simulink model "VCU_CS75_12_16_Test"  (R2014a)
settings: Solver=FixedStepDiscrete  StartTime=0.0  StopTime=25  FixedStep=0.0005  RelTol=1e-3
undefined symbols (not defined in the file): ecucoder_acal, I_SW01_L, LaterlAngleCommand, LDW, RemoteAcclPosition
libraries: simulink x913, ec5744lib x39
(part 5 of 30)

== system VCU_CS75_12_16_Test/长安CS75底盘程序，20ms一次/Input/DBC转化的messages（存底）/ReceiveMessages13/SAS_108 ==
  input : Inport
  Demux : Demux  Outputs=8
  SAS_CRCCheck_Ad : Sum
  SAS_CRCCheck_Convert : DataTypeConversion  OutDataTypeStr=uint32
  SAS_CRCCheck_F : Gain
  SAS_CRCCheck_L : simulink/Logic and Bit Operations/Bitwise Operator  logicop=AND  UseBitMask=on  BitMask=255  BitMaskRealWorld=Stored Integer
  SAS_CRCCheck_O : Constant  Value=0  OutDataTypeStr=single
  SAS_CRCCheck_S : ArithShift
  SAS_CRCCheck_Sub : Subsystem
  SAS_CRCCheck_sat : Saturate  UpperLimit=255  LowerLimit=0
  SAS_CRCCheckcv : DataTypeConversion
  SAS_Calibrated_Ad : Sum
  SAS_Calibrated_Convert : DataTypeConversion  OutDataTypeStr=uint32
  SAS_Calibrated_F : Gain
  SAS_Calibrated_L : simulink/Logic and Bit Operations/Bitwise Operator  logicop=AND  UseBitMask=on  BitMask=32  BitMaskRealWorld=Stored Integer
  SAS_Calibrated_O : Constant  Value=0  OutDataTypeStr=single
  SAS_Calibrated_S : ArithShift  BitShiftNumber=5
  SAS_Calibrated_Sub : Subsystem
  SAS_Calibrated_sat : Saturate  UpperLimit=1  LowerLimit=0
  SAS_Calibratedcv : DataTypeConversion
  SAS_RollingCounter_Ad : Sum
  SAS_RollingCounter_Convert : DataTypeConversion  OutDataTypeStr=uint32
  SAS_RollingCounter_F : Gain
  SAS_RollingCounter_L : simulink/Logic and Bit Operations/Bitwise Operator  logicop=AND  UseBitMask=on  BitMask=15  BitMaskRealWorld=Stored Integer
  SAS_RollingCounter_O : Constant  Value=0  OutDataTypeStr=single
  SAS_RollingCounter_S : ArithShift
  SAS_RollingCounter_Sub : Subsystem
  SAS_RollingCounter_sat : Saturate  UpperLimit=15  LowerLimit=0
  SAS_RollingCountercv : DataTypeConversion
  SAS_SASFailure_Ad : Sum
  SAS_SASFailure_Convert : DataTypeConversion  OutDataTypeStr=uint32
  SAS_SASFailure_F : Gain
  SAS_SASFailure_L : simulink/Logic and Bit Operations/Bitwise Operator  logicop=AND  UseBitMask=on  BitMask=64  BitMaskRealWorld=Stored Integer
  SAS_SASFailure_O : Constant  Value=0  OutDataTypeStr=single
  SAS_SASFailure_S : ArithShift  BitShiftNumber=6
  SAS_SASFailure_Sub : Subsystem
  SAS_SASFailure_sat : Saturate  UpperLimit=1  LowerLimit=0
  SAS_SASFailurecv : DataTypeConversion
  SAS_SteeringAngleCS : ArithShift  BitShiftNumber=-16
  SAS_SteeringAngleCS1 : ArithShift  BitShiftNumber=-15
  SAS_SteeringAngleConS : Constant  OutDataTypeStr=single
  SAS_SteeringAngleMinus : UnaryMinus
  SAS_SteeringAngleROP : RelationalOperator  OutDataTypeStr=boolean
  SAS_SteeringAngleSW : Switch  Criteria=u2 ~= 0
  SAS_SteeringAngleSpeed_Ad : Sum
  SAS_SteeringAngleSpeed_Convert : DataTypeConversion  OutDataTypeStr=uint32
  SAS_SteeringAngleSpeed_F : Gain  Gain=4
  SAS_SteeringAngleSpeed_L : simulink/Logic and Bit Operations/Bitwise Operator  logicop=AND  UseBitMask=on  BitMask=255  BitMaskRealWorld=Stored Integer
  SAS_SteeringAngleSpeed_O : Constant  Value=0  OutDataTypeStr=single
  SAS_SteeringAngleSpeed_S : ArithShift
  SAS_SteeringAngleSpeed_Sub : Subsystem
  SAS_SteeringAngleSpeed_sat : Saturate  UpperLimit=1020  LowerLimit=0
  SAS_SteeringAngleSpeedcv : DataTypeConversion
  SAS_SteeringAngleValid_Ad : Sum
  SAS_SteeringAngleValid_Convert : DataTypeConversion  OutDataTypeStr=uint32
  SAS_SteeringAngleValid_F : Gain
  SAS_SteeringAngleValid_L : simulink/Logic and Bit Operations/Bitwise Operator  logicop=AND  UseBitMask=on  BitMask=128  BitMaskRealWorld=Stored Integer
  SAS_SteeringAngleValid_O : Constant  Value=0  OutDataTypeStr=single
  SAS_SteeringAngleValid_S : ArithShift  BitShiftNumber=7
  SAS_SteeringAngleValid_Sub : Subsystem
  SAS_SteeringAngleValid_sat : Saturate  UpperLimit=1  LowerLimit=0
  SAS_SteeringAngleValidcv : DataTypeConversion
  SAS_SteeringAngle_Ad : Sum
  SAS_SteeringAngle_Convert : DataTypeConversion  OutDataTypeStr=uint32
  SAS_SteeringAngle_F : Gain  Gain=0.1
  SAS_SteeringAngle_L : simulink/Logic and Bit Operations/Bitwise Operator  logicop=AND  UseBitMask=on  BitMask=65535  BitMaskRealWorld=Stored Integer
  SAS_SteeringAngle_O : Constant  Value=0  OutDataTypeStr=single
  SAS_SteeringAngle_S : ArithShift
  SAS_SteeringAngle_Sub : Subsystem
  SAS_SteeringAngle_sat : Saturate  UpperLimit=780  LowerLimit=-780
  SAS_SteeringAnglecv : DataTypeConversion
  SAS_SteeringAngleinput1_Ad : Sum
  SAS_SteeringAngleinput1_C : Constant  Value=256
  SAS_SteeringAngleinput1_P : Product
  SAS_SteeringAnglesubcon : Sum  Inputs=+-
  SAS_SteeringAngle_Out : Outport
  SAS_SteeringAngleSpeed_Out : Outport  Port=2
  SAS_Calibrated_Out : Outport  Port=3
  SAS_SASFailure_Out : Outport  Port=4
  SAS_SteeringAngleValid_Out : Outport  Port=5
  SAS_RollingCounter_Out : Outport  Port=6
  SAS_CRCCheck_Out : Outport  Port=7
  wires:
  input/1 -> Demux/1
  SAS_CRCCheckcv/1 -> SAS_CRCCheck_F/1
  SAS_CRCCheck_S/1 -> SAS_CRCCheckcv/1
  SAS_CRCCheck_L/1 -> SAS_CRCCheck_S/1
  SAS_CRCCheck_Convert/1 -> SAS_CRCCheck_L/1
  SAS_CRCCheck_Sub/1(Out1) -> SAS_CRCCheck_Convert/1
  Demux/8 -> SAS_CRCCheck_Sub/1(In1)
  SAS_CRCCheck_sat/1 -> SAS_CRCCheck_Out/1
  SAS_CRCCheck_Ad/1 -> SAS_CRCCheck_sat/1
  SAS_CRCCheck_O/1 -> SAS_CRCCheck_Ad/2
  SAS_CRCCheck_F/1 -> SAS_CRCCheck_Ad/1
  SAS_RollingCountercv/1 -> SAS_RollingCounter_F/1
  SAS_RollingCounter_S/1 -> SAS_RollingCountercv/1
  SAS_RollingCounter_L/1 -> SAS_RollingCounter_S/1
  SAS_RollingCounter_Convert/1 -> SAS_RollingCounter_L/1
  SAS_RollingCounter_Sub/1(Out1) -> SAS_RollingCounter_Convert/1
  Demux/7 -> SAS_RollingCounter_Sub/1(In1)
  SAS_RollingCounter_sat/1 -> SAS_RollingCounter_Out/1
  SAS_RollingCounter_Ad/1 -> SAS_RollingCounter_sat/1
  SAS_RollingCounter_O/1 -> SAS_RollingCounter_Ad/2
  SAS_RollingCounter_F/1 -> SAS_RollingCounter_Ad/1
  SAS_SteeringAngleValidcv/1 -> SAS_SteeringAngleValid_F/1
  SAS_SteeringAngleValid_S/1 -> SAS_SteeringAngleValidcv/1
  SAS_SteeringAngleValid_L/1 -> SAS_SteeringAngleValid_S/1
  SAS_SteeringAngleValid_Convert/1 -> SAS_SteeringAngleValid_L/1
  SAS_SteeringAngleValid_Sub/1(Out1) -> SAS_SteeringAngleValid_Convert/1
  SAS_SteeringAngleValid_sat/1 -> SAS_SteeringAngleValid_Out/1
  SAS_SteeringAngleValid_Ad/1 -> SAS_SteeringAngleValid_sat/1
  SAS_SteeringAngleValid_O/1 -> SAS_SteeringAngleValid_Ad/2
  SAS_SteeringAngleValid_F/1 -> SAS_SteeringAngleValid_Ad/1
  SAS_SASFailurecv/1 -> SAS_SASFailure_F/1
  SAS_SASFailure_S/1 -> SAS_SASFailurecv/1
  SAS_SASFailure_L/1 -> SAS_SASFailure_S/1
  SAS_SASFailure_Convert/1 -> SAS_SASFailure_L/1
  SAS_SASFailure_Sub/1(Out1) -> SAS_SASFailure_Convert/1
  SAS_SASFailure_sat/1 -> SAS_SASFailure_Out/1
  SAS_SASFailure_Ad/1 -> SAS_SASFailure_sat/1
  SAS_SASFailure_O/1 -> SAS_SASFailure_Ad/2
  SAS_SASFailure_F/1 -> SAS_SASFailure_Ad/1
  SAS_Calibratedcv/1 -> SAS_Calibrated_F/1
  SAS_Calibrated_S/1 -> SAS_Calibratedcv/1
  SAS_Calibrated_L/1 -> SAS_Calibrated_S/1
  SAS_Calibrated_Convert/1 -> SAS_Calibrated_L/1
  SAS_Calibrated_Sub/1(Out1) -> SAS_Calibrated_Convert/1
  Demux/4 -> SAS_SteeringAngleValid_Sub/1(In1), SAS_SASFailure_Sub/1(In1), SAS_Calibrated_Sub/1(In1)
  SAS_Calibrated_sat/1 -> SAS_Calibrated_Out/1
  SAS_Calibrated_Ad/1 -> SAS_Calibrated_sat/1
  SAS_Calibrated_O/1 -> SAS_Calibrated_Ad/2
  SAS_Calibrated_F/1 -> SAS_Calibrated_Ad/1
  SAS_SteeringAngleSpeedcv/1 -> SAS_SteeringAngleSpeed_F/1
  SAS_SteeringAngleSpeed_S/1 -> SAS_SteeringAngleSpeedcv/1
  SAS_SteeringAngleSpeed_L/1 -> SAS_SteeringAngleSpeed_S/1
  SAS_SteeringAngleSpeed_Convert/1 -> SAS_SteeringAngleSpeed_L/1
  SAS_SteeringAngleSpeed_Sub/1(Out1) -> SAS_SteeringAngleSpeed_Convert/1
  Demux/3 -> SAS_SteeringAngleSpeed_Sub/1(In1)
  SAS_SteeringAngleSpeed_sat/1 -> SAS_SteeringAngleSpeed_Out/1
  SAS_SteeringAngleSpeed_Ad/1 -> SAS_SteeringAngleSpeed_sat/1
  SAS_SteeringAngleSpeed_O/1 -> SAS_SteeringAngleSpeed_Ad/2
  SAS_SteeringAngleSpeed_F/1 -> SAS_SteeringAngleSpeed_Ad/1
  SAS_SteeringAngleROP/1 -> SAS_SteeringAngleSW/2
  SAS_SteeringAngleSW/1 -> SAS_SteeringAngle_F/1
  SAS_SteeringAngleMinus/1 -> SAS_SteeringAngleSW/1
  SAS_SteeringAnglesubcon/1 -> SAS_SteeringAngleMinus/1
  SAS_SteeringAngleCS/1 -> SAS_SteeringAnglesubcon/1
  SAS_SteeringAngleCS1/1 -> SAS_SteeringAngleROP/2
  SAS_SteeringAngleConS/1 -> SAS_SteeringAngleCS1/1, SAS_SteeringAngleCS/1
  SAS_SteeringAnglecv/1 -> SAS_SteeringAngleSW/3, SAS_SteeringAnglesubcon/2, SAS_SteeringAngleROP/1
  SAS_SteeringAngle_S/1 -> SAS_SteeringAnglecv/1
  SAS_SteeringAngle_L/1 -> SAS_SteeringAngle_S/1
  SAS_SteeringAngle_Convert/1 -> SAS_SteeringAngle_L/1
  SAS_SteeringAngle_Sub/1(Out1) -> SAS_SteeringAngle_Convert/1
  SAS_SteeringAngleinput1_Ad/1 -> SAS_SteeringAngle_Sub/1(In1)
  Demux/2 -> SAS_SteeringAngleinput1_Ad/2
  SAS_SteeringAngleinput1_P/1 -> SAS_SteeringAngleinput1_Ad/1
  SAS_SteeringAngleinput1_C/1 -> SAS_SteeringAngleinput1_P/2
  Demux/1 -> SAS_SteeringAngleinput1_P/1
  SAS_SteeringAngle_sat/1 -> SAS_SteeringAngle_Out/1
  SAS_SteeringAngle_Ad/1 -> SAS_SteeringAngle_sat/1
  SAS_SteeringAngle_O/1 -> SAS_SteeringAngle_Ad/2
  SAS_SteeringAngle_F/1 -> SAS_SteeringAngle_Ad/1

== system VCU_CS75_12_16_Test/长安CS75底盘程序，20ms一次/Input/DBC转化的messages（存底）/ReceiveMessages14/SCM_3B8 ==
  input : Inport
  Demux : Demux  Outputs=8
  SCM_ACCCancel_Ad : Sum
  SCM_ACCCancel_Convert : DataTypeConversion  OutDataTypeStr=uint32
  SCM_ACCCancel_F : Gain
  SCM_ACCCancel_L : simulink/Logic and Bit Operations/Bitwise Operator  logicop=AND  UseBitMask=on  BitMask=4  BitMaskRealWorld=Stored Integer
  SCM_ACCCancel_O : Constant  Value=0  OutDataTypeStr=single
  SCM_ACCCancel_S : ArithShift  BitShiftNumber=2
  SCM_ACCCancel_Sub : Subsystem
  SCM_ACCCancel_sat : Saturate  UpperLimit=0  LowerLimit=0
  SCM_ACCCancelcv : DataTypeConversion
  SCM_ACCOn_Ad : Sum
  SCM_ACCOn_Convert : DataTypeConversion  OutDataTypeStr=uint32
  SCM_ACCOn_F : Gain
  SCM_ACCOn_L : simulink/Logic and Bit Operations/Bitwise Operator  logicop=AND  UseBitMask=on  BitMask=1  BitMaskRealWorld=Stored Integer
  SCM_ACCOn_O : Constant  Value=0  OutDataTypeStr=single
  SCM_ACCOn_S : ArithShift
  SCM_ACCOn_Sub : Subsystem
  SCM_ACCOn_sat : Saturate  UpperLimit=0  LowerLimit=0
  SCM_ACCOncv : DataTypeConversion
  SCM_IACCOn_Ad : Sum
  SCM_IACCOn_Convert : DataTypeConversion  OutDataTypeStr=uint32
  SCM_IACCOn_F : Gain
  SCM_IACCOn_L : simulink/Logic and Bit Operations/Bitwise Operator  logicop=AND  UseBitMask=on  BitMask=16  BitMaskRealWorld=Stored Integer
  SCM_IACCOn_O : Constant  Value=0  OutDataTypeStr=single
  SCM_IACCOn_S : ArithShift  BitShiftNumber=4
  SCM_IACCOn_Sub : Subsystem
  SCM_IACCOn_sat : Saturate  UpperLimit=0  LowerLimit=0
  SCM_IACCOncv : DataTypeConversion
  SCM_Resume_Ad : Sum
  SCM_Resume_Convert : DataTypeConversion  OutDataTypeStr=uint32
  SCM_Resume_F : Gain
  SCM_Resume_L : simulink/Logic and Bit Operations/Bitwise Operator  logicop=AND  UseBitMask=on  BitMask=16  BitMaskRealWorld=Stored Integer
  SCM_Resume_O : Constant  Value=0  OutDataTypeStr=single
  SCM_Resume_S : ArithShift  BitShiftNumber=4
  SCM_Resume_Sub : Subsystem
  SCM_Resume_sat : Saturate  UpperLimit=0  LowerLimit=0
  SCM_Resumecv : DataTypeConversion
  SCM_Speeddecrease_Ad : Sum
  SCM_Speeddecrease_Convert : DataTypeConversion  OutDataTypeStr=uint32
  SCM_Speeddecrease_F : Gain
  SCM_Speeddecrease_L : simulink/Logic and Bit Operations/Bitwise Operator  logicop=AND  UseBitMask=on  BitMask=64  BitMaskRealWorld=Stored Integer
  SCM_Speeddecrease_O : Constant  Value=0  OutDataTypeStr=single
  SCM_Speeddecrease_S : ArithShift  BitShiftNumber=6
  SCM_Speeddecrease_Sub : Subsystem
  SCM_Speeddecrease_sat : Saturate  UpperLimit=0  LowerLimit=0
  SCM_Speeddecreasecv : DataTypeConversion
  SCM_TimeGap_Ad : Sum
  SCM_TimeGap_Convert : DataTypeConversion  OutDataTypeStr=uint32
  SCM_TimeGap_F : Gain
  SCM_TimeGap_L : simulink/Logic and Bit Operations/Bitwise Operator  logicop=AND  UseBitMask=on  BitMask=1  BitMaskRealWorld=Stored Integer
  SCM_TimeGap_O : Constant  Value=0  OutDataTypeStr=single
  SCM_TimeGap_S : ArithShift
  SCM_TimeGap_Sub : Subsystem
  SCM_TimeGap_sat : Saturate  UpperLimit=0  LowerLimit=0
  SCM_TimeGapcv : DataTypeConversion
  SCM_ACCOn_Out : Outport
  SCM_ACCCancel_Out : Outport  Port=2
  SCM_Resume_Out : Outport  Port=3
  SCM_Speeddecrease_Out : Outport  Port=4
  SCM_TimeGap_Out : Outport  Port=5
  SCM_IACCOn_Out : Outport  Port=6
  wires:
  input/1 -> Demux/1
  SCM_IACCOncv/1 -> SCM_IACCOn_F/1
  SCM_IACCOn_S/1 -> SCM_IACCOncv/1
  SCM_IACCOn_L/1 -> SCM_IACCOn_S/1
  SCM_IACCOn_Convert/1 -> SCM_IACCOn_L/1
  SCM_IACCOn_Sub/1(Out1) -> SCM_IACCOn_Convert/1
  SCM_IACCOn_sat/1 -> SCM_IACCOn_Out/1
  SCM_IACCOn_Ad/1 -> SCM_IACCOn_sat/1
  SCM_IACCOn_O/1 -> SCM_IACCOn_Ad/2
  SCM_IACCOn_F/1 -> SCM_IACCOn_Ad/1
  SCM_TimeGapcv/1 -> SCM_TimeGap_F/1
  SCM_TimeGap_S/1 -> SCM_TimeGapcv/1
  SCM_TimeGap_L/1 -> SCM_TimeGap_S/1
  SCM_TimeGap_Convert/1 -> SCM_TimeGap_L/1
  SCM_TimeGap_Sub/1(Out1) -> SCM_TimeGap_Convert/1
  Demux/2 -> SCM_IACCOn_Sub/1(In1), SCM_TimeGap_Sub/1(In1)
  SCM_TimeGap_sat/1 -> SCM_TimeGap_Out/1
  SCM_TimeGap_Ad/1 -> SCM_TimeGap_sat/1
  SCM_TimeGap_O/1 -> SCM_TimeGap_Ad/2
  SCM_TimeGap_F/1 -> SCM_TimeGap_Ad/1
  SCM_Speeddecreasecv/1 -> SCM_Speeddecrease_F/1
  SCM_Speeddecrease_S/1 -> SCM_Speeddecreasecv/1
  SCM_Speeddecrease_L/1 -> SCM_Speeddecrease_S/1
  SCM_Speeddecrease_Convert/1 -> SCM_Speeddecrease_L/1
  SCM_Speeddecrease_Sub/1(Out1) -> SCM_Speeddecrease_Convert/1
  SCM_Speeddecrease_sat/1 -> SCM_Speeddecrease_Out/1
  SCM_Speeddecrease_Ad/1 -> SCM_Speeddecrease_sat/1
  SCM_Speeddecrease_O/1 -> SCM_Speeddecrease_Ad/2
  SCM_Speeddecrease_F/1 -> SCM_Speeddecrease_Ad/1
  SCM_Resumecv/1 -> SCM_Resume_F/1
  SCM_Resume_S/1 -> SCM_Resumecv/1
  SCM_Resume_L/1 -> SCM_Resume_S/1
  SCM_Resume_Convert/1 -> SCM_Resume_L/1
  SCM_Resume_Sub/1(Out1) -> SCM_Resume_Convert/1
  SCM_Resume_sat/1 -> SCM_Resume_Out/1
  SCM_Resume_Ad/1 -> SCM_Resume_sat/1
  SCM_Resume_O/1 -> SCM_Resume_Ad/2
  SCM_Resume_F/1 -> SCM_Resume_Ad/1
  SCM_ACCCancelcv/1 -> SCM_ACCCancel_F/1
  SCM_ACCCancel_S/1 -> SCM_ACCCancelcv/1
  SCM_ACCCancel_L/1 -> SCM_ACCCancel_S/1
  SCM_ACCCancel_Convert/1 -> SCM_ACCCancel_L/1
  SCM_ACCCancel_Sub/1(Out1) -> SCM_ACCCancel_Convert/1
  SCM_ACCCancel_sat/1 -> SCM_ACCCancel_Out/1
  SCM_ACCCancel_Ad/1 -> SCM_ACCCancel_sat/1
  SCM_ACCCancel_O/1 -> SCM_ACCCancel_Ad/2
  SCM_ACCCancel_F/1 -> SCM_ACCCancel_Ad/1
  SCM_ACCOncv/1 -> SCM_ACCOn_F/1
  SCM_ACCOn_S/1 -> SCM_ACCOncv/1
  SCM_ACCOn_L/1 -> SCM_ACCOn_S/1
  SCM_ACCOn_Convert/1 -> SCM_ACCOn_L/1
  SCM_ACCOn_Sub/1(Out1) -> SCM_ACCOn_Convert/1
  Demux/1 -> SCM_Speeddecrease_Sub/1(In1), SCM_Resume_Sub/1(In1), SCM_ACCCancel_Sub/1(In1), SCM_ACCOn_Sub/1(In1)
  SCM_ACCOn_sat/1 -> SCM_ACCOn_Out/1
  SCM_ACCOn_Ad/1 -> SCM_ACCOn_sat/1
  SCM_ACCOn_O/1 -> SCM_ACCOn_Ad/2
  SCM_ACCOn_F/1 -> SCM_ACCOn_Ad/1

== system VCU_CS75_12_16_Test/长安CS75底盘程序，20ms一次/Input/DBC转化的messages（存底）/ReceiveMessages15/SRS_005 ==
  input : Inport
  Demux : Demux  Outputs=8
  SRS_DriverBuckleSwitchStatus_Ad : Sum
  SRS_DriverBuckleSwitchStatus_Convert : DataTypeConversion  OutDataTypeStr=uint32
  SRS_DriverBuckleSwitchStatus_F : Gain
  SRS_DriverBuckleSwitchStatus_L : simulink/Logic and Bit Operations/Bitwise Operator  logicop=AND  UseBitMask=on  BitMask=192  BitMaskRealWorld=Stored Integer
  SRS_DriverBuckleSwitchStatus_O : Constant  Value=0  OutDataTypeStr=single
  SRS_DriverBuckleSwitchStatus_S : ArithShift  BitShiftNumber=6
  SRS_DriverBuckleSwitchStatus_Sub : Subsystem
  SRS_DriverBuckleSwitchStatus_sat : Saturate  UpperLimit=3  LowerLimit=0
  SRS_DriverBuckleSwitchStatuscv : DataTypeConversion
  SRS_RollingCounter_Ad : Sum
  SRS_RollingCounter_Convert : DataTypeConversion  OutDataTypeStr=uint32
  SRS_RollingCounter_F : Gain
  SRS_RollingCounter_L : simulink/Logic and Bit Operations/Bitwise Operator  logicop=AND  UseBitMask=on  BitMask=15  BitMaskRealWorld=Stored Integer
  SRS_RollingCounter_O : Constant  Value=0  OutDataTypeStr=single
  SRS_RollingCounter_S : ArithShift
  SRS_RollingCounter_Sub : Subsystem
  SRS_RollingCounter_sat : Saturate  UpperLimit=15  LowerLimit=0
  SRS_RollingCountercv : DataTypeConversion
  SRS_DriverBuckleSwitchStatus_Out : Outport
  SRS_RollingCounter_Out : Outport  Port=2
  wires:
  input/1 -> Demux/1
  SRS_RollingCountercv/1 -> SRS_RollingCounter_F/1
  SRS_RollingCounter_S/1 -> SRS_RollingCountercv/1
  SRS_RollingCounter_L/1 -> SRS_RollingCounter_S/1
  SRS_RollingCounter_Convert/1 -> SRS_RollingCounter_L/1
  SRS_RollingCounter_Sub/1(Out1) -> SRS_RollingCounter_Convert/1
  Demux/4 -> SRS_RollingCounter_Sub/1(In1)
  SRS_RollingCounter_sat/1 -> SRS_RollingCounter_Out/1
  SRS_RollingCounter_Ad/1 -> SRS_RollingCounter_sat/1
  SRS_RollingCounter_O/1 -> SRS_RollingCounter_Ad/2
  SRS_RollingCounter_F/1 -> SRS_RollingCounter_Ad/1
  SRS_DriverBuckleSwitchStatuscv/1 -> SRS_DriverBuckleSwitchStatus_F/1
  SRS_DriverBuckleSwitchStatus_S/1 -> SRS_DriverBuckleSwitchStatuscv/1
  SRS_DriverBuckleSwitchStatus_L/1 -> SRS_DriverBuckleSwitchStatus_S/1
  SRS_DriverBuckleSwitchStatus_Convert/1 -> SRS_DriverBuckleSwitchStatus_L/1
  SRS_DriverBuckleSwitchStatus_Sub/1(Out1) -> SRS_DriverBuckleSwitchStatus_Convert/1
  Demux/2 -> SRS_DriverBuckleSwitchStatus_Sub/1(In1)
  SRS_DriverBuckleSwitchStatus_sat/1 -> SRS_DriverBuckleSwitchStatus_Out/1
  SRS_DriverBuckleSwitchStatus_Ad/1 -> SRS_DriverBuckleSwitchStatus_sat/1
  SRS_DriverBuckleSwitchStatus_O/1 -> SRS_DriverBuckleSwitchStatus_Ad/2
  SRS_DriverBuckleSwitchStatus_F/1 -> SRS_DriverBuckleSwitchStatus_Ad/1

== system VCU_CS75_12_16_Test/长安CS75底盘程序，20ms一次/Input/DBC转化的messages（存底）/ReceiveMessages16/TCU_286 ==
  input : Inport
  Demux : Demux  Outputs=8
  TCU_ActualGearValid_Ad : Sum
  TCU_ActualGearValid_Convert : DataTypeConversion  OutDataTypeStr=uint32
  TCU_ActualGearValid_F : Gain
  TCU_ActualGearValid_L : simulink/Logic and Bit Operations/Bitwise Operator  logicop=AND  UseBitMask=on  BitMask=32  BitMaskRealWorld=Stored Integer
  TCU_ActualGearValid_O : Constant  Value=0  OutDataTypeStr=single
  TCU_ActualGearValid_S : ArithShift  BitShiftNumber=5
  TCU_ActualGearValid_Sub : Subsystem
  TCU_ActualGearValid_sat : Saturate  UpperLimit=1  LowerLimit=0
  TCU_ActualGearValidcv : DataTypeConversion
  TCU_ActualGear_Ad : Sum
  TCU_ActualGear_Convert : DataTypeConversion  OutDataTypeStr=uint32
  TCU_ActualGear_F : Gain
  TCU_ActualGear_L : simulink/Logic and Bit Operations/Bitwise Operator  logicop=AND  UseBitMask=on  BitMask=15  BitMaskRealWorld=Stored Integer
  TCU_ActualGear_O : Constant  Value=0  OutDataTypeStr=single
  TCU_ActualGear_S : ArithShift
  TCU_ActualGear_Sub : Subsystem
  TCU_ActualGear_sat : Saturate  UpperLimit=15  LowerLimit=0
  TCU_ActualGearcv : DataTypeConversion
  TCU_GearShiftPosition_Ad : Sum
  TCU_GearShiftPosition_Convert : DataTypeConversion  OutDataTypeStr=uint32
  TCU_GearShiftPosition_F : Gain
  TCU_GearShiftPosition_L : simulink/Logic and Bit Operations/Bitwise Operator  logicop=AND  UseBitMask=on  BitMask=240  BitMaskRealWorld=Stored Integer
  TCU_GearShiftPosition_O : Constant  Value=0  OutDataTypeStr=single
  TCU_GearShiftPosition_S : ArithShift  BitShiftNumber=4
  TCU_GearShiftPosition_Sub : Subsystem
  TCU_GearShiftPosition_sat : Saturate  UpperLimit=15  LowerLimit=0
  TCU_GearShiftPositioncv : DataTypeConversion
  TCU_ShiftPositionValid_Ad : Sum
  TCU_ShiftPositionValid_Convert : DataTypeConversion  OutDataTypeStr=uint32
  TCU_ShiftPositionValid_F : Gain
  TCU_ShiftPositionValid_L : simulink/Logic and Bit Operations/Bitwise Operator  logicop=AND  UseBitMask=on  BitMask=16  BitMaskRealWorld=Stored Integer
  TCU_ShiftPositionValid_O : Constant  Value=0  OutDataTypeStr=single
  TCU_ShiftPositionValid_S : ArithShift  BitShiftNumber=4
  TCU_ShiftPositionValid_Sub : Subsystem
  TCU_ShiftPositionValid_sat : Saturate  UpperLimit=1  LowerLimit=0
  TCU_ShiftPositionValidcv : DataTypeConversion
  TCU_ActualGear_Out : Outport
  TCU_ShiftPositionValid_Out : Outport  Port=2
  TCU_ActualGearValid_Out : Outport  Port=3
  TCU_GearShiftPosition_Out : Outport  Port=4
  wires:
  input/1 -> Demux/1
  TCU_GearShiftPositioncv/1 -> TCU_GearShiftPosition_F/1
  TCU_GearShiftPosition_S/1 -> TCU_GearShiftPositioncv/1
  TCU_GearShiftPosition_L/1 -> TCU_GearShiftPosition_S/1
  TCU_GearShiftPosition_Convert/1 -> TCU_GearShiftPosition_L/1
  TCU_GearShiftPosition_Sub/1(Out1) -> TCU_GearShiftPosition_Convert/1
  Demux/3 -> TCU_GearShiftPosition_Sub/1(In1)
  TCU_GearShiftPosition_sat/1 -> TCU_GearShiftPosition_Out/1
  TCU_GearShiftPosition_Ad/1 -> TCU_GearShiftPosition_sat/1
  TCU_GearShiftPosition_O/1 -> TCU_GearShiftPosition_Ad/2
  TCU_GearShiftPosition_F/1 -> TCU_GearShiftPosition_Ad/1
  TCU_ActualGearValidcv/1 -> TCU_ActualGearValid_F/1
  TCU_ActualGearValid_S/1 -> TCU_ActualGearValidcv/1
  TCU_ActualGearValid_L/1 -> TCU_ActualGearValid_S/1
  TCU_ActualGearValid_Convert/1 -> TCU_ActualGearValid_L/1
  TCU_ActualGearValid_Sub/1(Out1) -> TCU_ActualGearValid_Convert/1
  TCU_ActualGearValid_sat/1 -> TCU_ActualGearValid_Out/1
  TCU_ActualGearValid_Ad/1 -> TCU_ActualGearValid_sat/1
  TCU_ActualGearValid_O/1 -> TCU_ActualGearValid_Ad/2
  TCU_ActualGearValid_F/1 -> TCU_ActualGearValid_Ad/1
  TCU_ShiftPositionValidcv/1 -> TCU_ShiftPositionValid_F/1
  TCU_ShiftPositionValid_S/1 -> TCU_ShiftPositionValidcv/1
  TCU_ShiftPositionValid_L/1 -> TCU_ShiftPositionValid_S/1
  TCU_ShiftPositionValid_Convert/1 -> TCU_ShiftPositionValid_L/1
  TCU_ShiftPositionValid_Sub/1(Out1) -> TCU_ShiftPositionValid_Convert/1
  TCU_ShiftPositionValid_sat/1 -> TCU_ShiftPositionValid_Out/1
  TCU_ShiftPositionValid_Ad/1 -> TCU_ShiftPositionValid_sat/1
  TCU_ShiftPositionValid_O/1 -> TCU_ShiftPositionValid_Ad/2
  TCU_ShiftPositionValid_F/1 -> TCU_ShiftPositionValid_Ad/1
  TCU_ActualGearcv/1 -> TCU_ActualGear_F/1
  TCU_ActualGear_S/1 -> TCU_ActualGearcv/1
  TCU_ActualGear_L/1 -> TCU_ActualGear_S/1
  TCU_ActualGear_Convert/1 -> TCU_ActualGear_L/1
  TCU_ActualGear_Sub/1(Out1) -> TCU_ActualGear_Convert/1
  Demux/2 -> TCU_ActualGearValid_Sub/1(In1), TCU_ShiftPositionValid_Sub/1(In1), TCU_ActualGear_Sub/1(In1)
  TCU_ActualGear_sat/1 -> TCU_ActualGear_Out/1
  TCU_ActualGear_Ad/1 -> TCU_ActualGear_sat/1
  TCU_ActualGear_O/1 -> TCU_ActualGear_Ad/2
  TCU_ActualGear_F/1 -> TCU_ActualGear_Ad/1

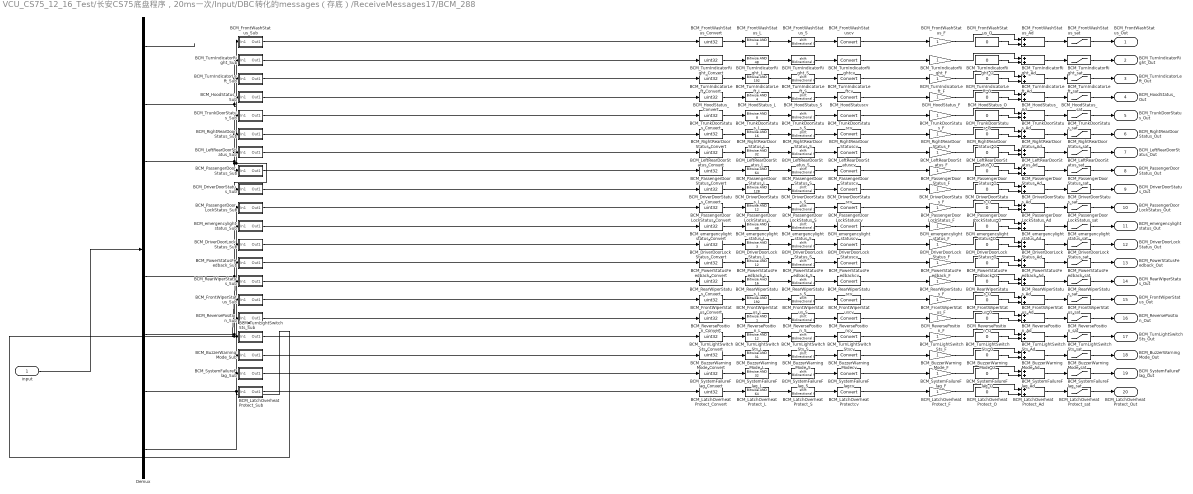
== system VCU_CS75_12_16_Test/长安CS75底盘程序，20ms一次/Input/DBC转化的messages（存底）/ReceiveMessages17/BCM_288 ==
  input : Inport
  BCM_BuzzerWarningMode_Ad : Sum
  BCM_BuzzerWarningMode_Convert : DataTypeConversion  OutDataTypeStr=uint32
  BCM_BuzzerWarningMode_F : Gain
  BCM_BuzzerWarningMode_L : simulink/Logic and Bit Operations/Bitwise Operator  logicop=AND  UseBitMask=on  BitMask=31  BitMaskRealWorld=Stored Integer
  BCM_BuzzerWarningMode_O : Constant  Value=0  OutDataTypeStr=single
  BCM_BuzzerWarningMode_S : ArithShift
  BCM_BuzzerWarningMode_Sub : Subsystem
  BCM_BuzzerWarningMode_sat : Saturate  UpperLimit=31  LowerLimit=0
  BCM_BuzzerWarningModecv : DataTypeConversion
  BCM_DriverDoorLockStatus_Ad : Sum
  BCM_DriverDoorLockStatus_Convert : DataTypeConversion  OutDataTypeStr=uint32
  BCM_DriverDoorLockStatus_F : Gain
  BCM_DriverDoorLockStatus_L : simulink/Logic and Bit Operations/Bitwise Operator  logicop=AND  UseBitMask=on  BitMask=3  BitMaskRealWorld=Stored Integer
  BCM_DriverDoorLockStatus_O : Constant  Value=0  OutDataTypeStr=single
  BCM_DriverDoorLockStatus_S : ArithShift
  BCM_DriverDoorLockStatus_Sub : Subsystem
  BCM_DriverDoorLockStatus_sat : Saturate  UpperLimit=3  LowerLimit=0
  BCM_DriverDoorLockStatuscv : DataTypeConversion
  BCM_DriverDoorStatus_Ad : Sum
  BCM_DriverDoorStatus_Convert : DataTypeConversion  OutDataTypeStr=uint32
  BCM_DriverDoorStatus_F : Gain
  BCM_DriverDoorStatus_L : simulink/Logic and Bit Operations/Bitwise Operator  logicop=AND  UseBitMask=on  BitMask=128  BitMaskRealWorld=Stored Integer
  BCM_DriverDoorStatus_O : Constant  Value=0  OutDataTypeStr=single
  BCM_DriverDoorStatus_S : ArithShift  BitShiftNumber=7
  BCM_DriverDoorStatus_Sub : Subsystem
  BCM_DriverDoorStatus_sat : Saturate  UpperLimit=1  LowerLimit=0
  BCM_DriverDoorStatuscv : DataTypeConversion
  BCM_FrontWashStatus_Ad : Sum
  BCM_FrontWashStatus_Convert : DataTypeConversion  OutDataTypeStr=uint32
  BCM_FrontWashStatus_F : Gain
  BCM_FrontWashStatus_L : simulink/Logic and Bit Operations/Bitwise Operator  logicop=AND  UseBitMask=on  BitMask=3  BitMaskRealWorld=Stored Integer
  BCM_FrontWashStatus_O : Constant  Value=0  OutDataTypeStr=single
  BCM_FrontWashStatus_S : ArithShift
  BCM_FrontWashStatus_Sub : Subsystem
  BCM_FrontWashStatus_sat : Saturate  UpperLimit=3  LowerLimit=0
  BCM_FrontWashStatuscv : DataTypeConversion
  BCM_FrontWiperStatus_Ad : Sum
  BCM_FrontWiperStatus_Convert : DataTypeConversion  OutDataTypeStr=uint32
  BCM_FrontWiperStatus_F : Gain
  BCM_FrontWiperStatus_L : simulink/Logic and Bit Operations/Bitwise Operator  logicop=AND  UseBitMask=on  BitMask=192  BitMaskRealWorld=Stored Integer
  BCM_FrontWiperStatus_O : Constant  Value=0  OutDataTypeStr=single
  BCM_FrontWiperStatus_S : ArithShift  BitShiftNumber=6
  BCM_FrontWiperStatus_Sub : Subsystem
  BCM_FrontWiperStatus_sat : Saturate  UpperLimit=3  LowerLimit=0
  BCM_FrontWiperStatuscv : DataTypeConversion
  BCM_HoodStatus_Ad : Sum
  BCM_HoodStatus_Convert : DataTypeConversion  OutDataTypeStr=uint32
  BCM_HoodStatus_F : Gain
  BCM_HoodStatus_L : simulink/Logic and Bit Operations/Bitwise Operator  logicop=AND  UseBitMask=on  BitMask=4  BitMaskRealWorld=Stored Integer
  BCM_HoodStatus_O : Constant  Value=0  OutDataTypeStr=single
  BCM_HoodStatus_S : ArithShift  BitShiftNumber=2
  BCM_HoodStatus_Sub : Subsystem
  BCM_HoodStatus_sat : Saturate  UpperLimit=1  LowerLimit=0
  BCM_HoodStatuscv : DataTypeConversion
  BCM_LatchOverheatProtect_Ad : Sum
  BCM_LatchOverheatProtect_Convert : DataTypeConversion  OutDataTypeStr=uint32
  BCM_LatchOverheatProtect_F : Gain
  BCM_LatchOverheatProtect_L : simulink/Logic and Bit Operations/Bitwise Operator  logicop=AND  UseBitMask=on  BitMask=64  BitMaskRealWorld=Stored Integer
  BCM_LatchOverheatProtect_O : Constant  Value=0  OutDataTypeStr=single
  BCM_LatchOverheatProtect_S : ArithShift  BitShiftNumber=6
  BCM_LatchOverheatProtect_Sub : Subsystem
  BCM_LatchOverheatProtect_sat : Saturate  UpperLimit=1  LowerLimit=0
  BCM_LatchOverheatProtectcv : DataTypeConversion
  BCM_LeftRearDoorStatus_Ad : Sum
  BCM_LeftRearDoorStatus_Convert : DataTypeConversion  OutDataTypeStr=uint32
  BCM_LeftRearDoorStatus_F : Gain
  BCM_LeftRearDoorStatus_L : simulink/Logic and Bit Operations/Bitwise Operator  logicop=AND  UseBitMask=on  BitMask=32  BitMaskRealWorld=Stored Integer
  BCM_LeftRearDoorStatus_O : Constant  Value=0  OutDataTypeStr=single
  BCM_LeftRearDoorStatus_S : ArithShift  BitShiftNumber=5
  BCM_LeftRearDoorStatus_Sub : Subsystem
  BCM_LeftRearDoorStatus_sat : Saturate  UpperLimit=1  LowerLimit=0
  BCM_LeftRearDoorStatuscv : DataTypeConversion
  BCM_PassengerDoorLockStatus_Ad : Sum
  BCM_PassengerDoorLockStatus_Convert : DataTypeConversion  OutDataTypeStr=uint32
  BCM_PassengerDoorLockStatus_F : Gain
  BCM_PassengerDoorLockStatus_L : simulink/Logic and Bit Operations/Bitwise Operator  logicop=AND  UseBitMask=on  BitMask=12  BitMaskRealWorld=Stored Integer
  BCM_PassengerDoorLockStatus_O : Constant  Value=0  OutDataTypeStr=single
  BCM_PassengerDoorLockStatus_S : ArithShift  BitShiftNumber=2
  BCM_PassengerDoorLockStatus_Sub : Subsystem
  BCM_PassengerDoorLockStatus_sat : Saturate  UpperLimit=3  LowerLimit=0
  BCM_PassengerDoorLockStatuscv : DataTypeConversion
  BCM_PassengerDoorStatus_Ad : Sum
  BCM_PassengerDoorStatus_Convert : DataTypeConversion  OutDataTypeStr=uint32
  BCM_PassengerDoorStatus_F : Gain
  BCM_PassengerDoorStatus_L : simulink/Logic and Bit Operations/Bitwise Operator  logicop=AND  UseBitMask=on  BitMask=64  BitMaskRealWorld=Stored Integer
  BCM_PassengerDoorStatus_O : Constant  Value=0  OutDataTypeStr=single
  BCM_PassengerDoorStatus_S : ArithShift  BitShiftNumber=6
  BCM_PassengerDoorStatus_Sub : Subsystem
  BCM_PassengerDoorStatus_sat : Saturate  UpperLimit=1  LowerLimit=0
  BCM_PassengerDoorStatuscv : DataTypeConversion
  BCM_PowerStatusFeedback_Ad : Sum
  BCM_PowerStatusFeedback_Convert : DataTypeConversion  OutDataTypeStr=uint32
  BCM_PowerStatusFeedback_F : Gain
  BCM_PowerStatusFeedback_L : simulink/Logic and Bit Operations/Bitwise Operator  logicop=AND  UseBitMask=on  BitMask=12  BitMaskRealWorld=Stored Integer
  BCM_PowerStatusFeedback_O : Constant  Value=0  OutDataTypeStr=single
  BCM_PowerStatusFeedback_S : ArithShift  BitShiftNumber=2
  BCM_PowerStatusFeedback_Sub : Subsystem
  BCM_PowerStatusFeedback_sat : Saturate  UpperLimit=3  LowerLimit=0
  BCM_PowerStatusFeedbackcv : DataTypeConversion
  BCM_RearWiperStatus_Ad : Sum
  BCM_RearWiperStatus_Convert : DataTypeConversion  OutDataTypeStr=uint32
  BCM_RearWiperStatus_F : Gain
  BCM_RearWiperStatus_L : simulink/Logic and Bit Operations/Bitwise Operator  logicop=AND  UseBitMask=on  BitMask=16  BitMaskRealWorld=Stored Integer
  BCM_RearWiperStatus_O : Constant  Value=0  OutDataTypeStr=single
  BCM_RearWiperStatus_S : ArithShift  BitShiftNumber=4
  BCM_RearWiperStatus_Sub : Subsystem
  BCM_RearWiperStatus_sat : Saturate  UpperLimit=1  LowerLimit=0
  BCM_RearWiperStatuscv : DataTypeConversion
  BCM_ReversePosition_Ad : Sum
  BCM_ReversePosition_Convert : DataTypeConversion  OutDataTypeStr=uint32
  BCM_ReversePosition_F : Gain
  BCM_ReversePosition_L : simulink/Logic and Bit Operations/Bitwise Operator  logicop=AND  UseBitMask=on  BitMask=1  BitMaskRealWorld=Stored Integer
  BCM_ReversePosition_O : Constant  Value=0  OutDataTypeStr=single
  BCM_ReversePosition_S : ArithShift
  BCM_ReversePosition_Sub : Subsystem
  BCM_ReversePosition_sat : Saturate  UpperLimit=1  LowerLimit=0
  BCM_ReversePositioncv : DataTypeConversion
  BCM_RightRearDoorStatus_Ad : Sum
  BCM_RightRearDoorStatus_Convert : DataTypeConversion  OutDataTypeStr=uint32
  BCM_RightRearDoorStatus_F : Gain
  BCM_RightRearDoorStatus_L : simulink/Logic and Bit Operations/Bitwise Operator  logicop=AND  UseBitMask=on  BitMask=16  BitMaskRealWorld=Stored Integer
  BCM_RightRearDoorStatus_O : Constant  Value=0  OutDataTypeStr=single
  BCM_RightRearDoorStatus_S : ArithShift  BitShiftNumber=4
  BCM_RightRearDoorStatus_Sub : Subsystem
  BCM_RightRearDoorStatus_sat : Saturate  UpperLimit=1  LowerLimit=0
  BCM_RightRearDoorStatuscv : DataTypeConversion
  BCM_SystemFailureFlag_Ad : Sum
  BCM_SystemFailureFlag_Convert : DataTypeConversion  OutDataTypeStr=uint32
  BCM_SystemFailureFlag_F : Gain
  BCM_SystemFailureFlag_L : simulink/Logic and Bit Operations/Bitwise Operator  logicop=AND  UseBitMask=on  BitMask=32  BitMaskRealWorld=Stored Integer
  BCM_SystemFailureFlag_O : Constant  Value=0  OutDataTypeStr=single
  BCM_SystemFailureFlag_S : ArithShift  BitShiftNumber=5
  BCM_SystemFailureFlag_Sub : Subsystem
  BCM_SystemFailureFlag_sat : Saturate  UpperLimit=1  LowerLimit=0
  BCM_SystemFailureFlagcv : DataTypeConversion
  BCM_TrunkDoorStatus_Ad : Sum
  BCM_TrunkDoorStatus_Convert : DataTypeConversion  OutDataTypeStr=uint32
  BCM_TrunkDoorStatus_F : Gain
  BCM_TrunkDoorStatus_L : simulink/Logic and Bit Operations/Bitwise Operator  logicop=AND  UseBitMask=on  BitMask=8  BitMaskRealWorld=Stored Integer
  BCM_TrunkDoorStatus_O : Constant  Value=0  OutDataTypeStr=single
  BCM_TrunkDoorStatus_S : ArithShift  BitShiftNumber=3
  BCM_TrunkDoorStatus_Sub : Subsystem
  BCM_TrunkDoorStatus_sat : Saturate  UpperLimit=1  LowerLimit=0
  BCM_TrunkDoorStatuscv : DataTypeConversion
  BCM_TurnIndicatorLeft_Ad : Sum
  BCM_TurnIndicatorLeft_Convert : DataTypeConversion  OutDataTypeStr=uint32
  BCM_TurnIndicatorLeft_F : Gain
  BCM_TurnIndicatorLeft_L : simulink/Logic and Bit Operations/Bitwise Operator  logicop=AND  UseBitMask=on  BitMask=192  BitMaskRealWorld=Stored Integer
  BCM_TurnIndicatorLeft_O : Constant  Value=0  OutDataTypeStr=single
  BCM_TurnIndicatorLeft_S : ArithShift  BitShiftNumber=6
  BCM_TurnIndicatorLeft_Sub : Subsystem
  BCM_TurnIndicatorLeft_sat : Saturate  UpperLimit=3  LowerLimit=0
  BCM_TurnIndicatorLeftcv : DataTypeConversion
  BCM_TurnIndicatorRight_Ad : Sum
  BCM_TurnIndicatorRight_Convert : DataTypeConversion  OutDataTypeStr=uint32
  BCM_TurnIndicatorRight_F : Gain
  BCM_TurnIndicatorRight_L : simulink/Logic and Bit Operations/Bitwise Operator  logicop=AND  UseBitMask=on  BitMask=48  BitMaskRealWorld=Stored Integer
  BCM_TurnIndicatorRight_O : Constant  Value=0  OutDataTypeStr=single
  BCM_TurnIndicatorRight_S : ArithShift  BitShiftNumber=4
  BCM_TurnIndicatorRight_Sub : Subsystem
  BCM_TurnIndicatorRight_sat : Saturate  UpperLimit=3  LowerLimit=0
  BCM_TurnIndicatorRightcv : DataTypeConversion
  BCM_TurnLightSwitchSts_Ad : Sum
  BCM_TurnLightSwitchSts_Convert : DataTypeConversion  OutDataTypeStr=uint32
  BCM_TurnLightSwitchSts_F : Gain
  BCM_TurnLightSwitchSts_L : simulink/Logic and Bit Operations/Bitwise Operator  logicop=AND  UseBitMask=on  BitMask=12  BitMaskRealWorld=Stored Integer
  BCM_TurnLightSwitchSts_O : Constant  Value=0  OutDataTypeStr=single
  BCM_TurnLightSwitchSts_S : ArithShift  BitShiftNumber=2
  BCM_TurnLightSwitchSts_Sub : Subsystem
  BCM_TurnLightSwitchSts_sat : Saturate  UpperLimit=3  LowerLimit=0
  BCM_TurnLightSwitchStscv : DataTypeConversion
  BCM_emergencylightstatus_Ad : Sum
  BCM_emergencylightstatus_Convert : DataTypeConversion  OutDataTypeStr=uint32
  BCM_emergencylightstatus_F : Gain
  BCM_emergencylightstatus_L : simulink/Logic and Bit Operations/Bitwise Operator  logicop=AND  UseBitMask=on  BitMask=48  BitMaskRealWorld=Stored Integer
  BCM_emergencylightstatus_O : Constant  Value=0  OutDataTypeStr=single
  BCM_emergencylightstatus_S : ArithShift  BitShiftNumber=4
  BCM_emergencylightstatus_Sub : Subsystem
  BCM_emergencylightstatus_sat : Saturate  UpperLimit=3  LowerLimit=0
  BCM_emergencylightstatuscv : DataTypeConversion
  Demux : Demux  Outputs=8
  BCM_FrontWashStatus_Out : Outport
  BCM_TurnIndicatorRight_Out : Outport  Port=2
  BCM_TurnIndicatorLeft_Out : Outport  Port=3
  BCM_HoodStatus_Out : Outport  Port=4
  BCM_TrunkDoorStatus_Out : Outport  Port=5
  BCM_RightRearDoorStatus_Out : Outport  Port=6
  BCM_LeftRearDoorStatus_Out : Outport  Port=7
  BCM_PassengerDoorStatus_Out : Outport  Port=8
  BCM_DriverDoorStatus_Out : Outport  Port=9
  BCM_PassengerDoorLockStatus_Out : Outport  Port=10
  BCM_emergencylightstatus_Out : Outport  Port=11
  BCM_DriverDoorLockStatus_Out : Outport  Port=12
  BCM_PowerStatusFeedback_Out : Outport  Port=13
  BCM_RearWiperStatus_Out : Outport  Port=14
  BCM_FrontWiperStatus_Out : Outport  Port=15
  BCM_ReversePosition_Out : Outport  Port=16
  BCM_TurnLightSwitchSts_Out : Outport  Port=17
  BCM_BuzzerWarningMode_Out : Outport  Port=18
  BCM_SystemFailureFlag_Out : Outport  Port=19
  BCM_LatchOverheatProtect_Out : Outport  Port=20
  wires:
  input/1 -> Demux/1
  BCM_LatchOverheatProtectcv/1 -> BCM_LatchOverheatProtect_F/1
  BCM_LatchOverheatProtect_S/1 -> BCM_LatchOverheatProtectcv/1
  BCM_LatchOverheatProtect_L/1 -> BCM_LatchOverheatProtect_S/1
  BCM_LatchOverheatProtect_Convert/1 -> BCM_LatchOverheatProtect_L/1
  BCM_LatchOverheatProtect_Sub/1(Out1) -> BCM_LatchOverheatProtect_Convert/1
  BCM_LatchOverheatProtect_sat/1 -> BCM_LatchOverheatProtect_Out/1
  BCM_LatchOverheatProtect_Ad/1 -> BCM_LatchOverheatProtect_sat/1
  BCM_LatchOverheatProtect_O/1 -> BCM_LatchOverheatProtect_Ad/2
  BCM_LatchOverheatProtect_F/1 -> BCM_LatchOverheatProtect_Ad/1
  BCM_SystemFailureFlagcv/1 -> BCM_SystemFailureFlag_F/1
  BCM_SystemFailureFlag_S/1 -> BCM_SystemFailureFlagcv/1
  BCM_SystemFailureFlag_L/1 -> BCM_SystemFailureFlag_S/1
  BCM_SystemFailureFlag_Convert/1 -> BCM_SystemFailureFlag_L/1
  BCM_SystemFailureFlag_Sub/1(Out1) -> BCM_SystemFailureFlag_Convert/1
  BCM_SystemFailureFlag_sat/1 -> BCM_SystemFailureFlag_Out/1
  BCM_SystemFailureFlag_Ad/1 -> BCM_SystemFailureFlag_sat/1
  BCM_SystemFailureFlag_O/1 -> BCM_SystemFailureFlag_Ad/2
  BCM_SystemFailureFlag_F/1 -> BCM_SystemFailureFlag_Ad/1
  BCM_BuzzerWarningModecv/1 -> BCM_BuzzerWarningMode_F/1
  BCM_BuzzerWarningMode_S/1 -> BCM_BuzzerWarningModecv/1
  BCM_BuzzerWarningMode_L/1 -> BCM_BuzzerWarningMode_S/1
  BCM_BuzzerWarningMode_Convert/1 -> BCM_BuzzerWarningMode_L/1
  BCM_BuzzerWarningMode_Sub/1(Out1) -> BCM_BuzzerWarningMode_Convert/1
  Demux/8 -> BCM_SystemFailureFlag_Sub/1(In1), BCM_BuzzerWarningMode_Sub/1(In1), BCM_LatchOverheatProtect_Sub/1(In1)
  BCM_BuzzerWarningMode_sat/1 -> BCM_BuzzerWarningMode_Out/1
  BCM_BuzzerWarningMode_Ad/1 -> BCM_BuzzerWarningMode_sat/1
  BCM_BuzzerWarningMode_O/1 -> BCM_BuzzerWarningMode_Ad/2
  BCM_BuzzerWarningMode_F/1 -> BCM_BuzzerWarningMode_Ad/1
  BCM_TurnLightSwitchStscv/1 -> BCM_TurnLightSwitchSts_F/1
  BCM_TurnLightSwitchSts_S/1 -> BCM_TurnLightSwitchStscv/1
  BCM_TurnLightSwitchSts_L/1 -> BCM_TurnLightSwitchSts_S/1
  BCM_TurnLightSwitchSts_Convert/1 -> BCM_TurnLightSwitchSts_L/1
  BCM_TurnLightSwitchSts_Sub/1(Out1) -> BCM_TurnLightSwitchSts_Convert/1
  BCM_TurnLightSwitchSts_sat/1 -> BCM_TurnLightSwitchSts_Out/1
  BCM_TurnLightSwitchSts_Ad/1 -> BCM_TurnLightSwitchSts_sat/1
  BCM_TurnLightSwitchSts_O/1 -> BCM_TurnLightSwitchSts_Ad/2
  BCM_TurnLightSwitchSts_F/1 -> BCM_TurnLightSwitchSts_Ad/1
  BCM_ReversePositioncv/1 -> BCM_ReversePosition_F/1
  BCM_ReversePosition_S/1 -> BCM_ReversePositioncv/1
  BCM_ReversePosition_L/1 -> BCM_ReversePosition_S/1
  BCM_ReversePosition_Convert/1 -> BCM_ReversePosition_L/1
  BCM_ReversePosition_Sub/1(Out1) -> BCM_ReversePosition_Convert/1
  Demux/7 -> BCM_TurnLightSwitchSts_Sub/1(In1), BCM_ReversePosition_Sub/1(In1)
  BCM_ReversePosition_sat/1 -> BCM_ReversePosition_Out/1
  BCM_ReversePosition_Ad/1 -> BCM_ReversePosition_sat/1
  BCM_ReversePosition_O/1 -> BCM_ReversePosition_Ad/2
  BCM_ReversePosition_F/1 -> BCM_ReversePosition_Ad/1
  BCM_FrontWiperStatuscv/1 -> BCM_FrontWiperStatus_F/1
  BCM_FrontWiperStatus_S/1 -> BCM_FrontWiperStatuscv/1
  BCM_FrontWiperStatus_L/1 -> BCM_FrontWiperStatus_S/1
  BCM_FrontWiperStatus_Convert/1 -> BCM_FrontWiperStatus_L/1
  BCM_FrontWiperStatus_Sub/1(Out1) -> BCM_FrontWiperStatus_Convert/1
  BCM_FrontWiperStatus_sat/1 -> BCM_FrontWiperStatus_Out/1
  BCM_FrontWiperStatus_Ad/1 -> BCM_FrontWiperStatus_sat/1
  BCM_FrontWiperStatus_O/1 -> BCM_FrontWiperStatus_Ad/2
  BCM_FrontWiperStatus_F/1 -> BCM_FrontWiperStatus_Ad/1
  BCM_RearWiperStatuscv/1 -> BCM_RearWiperStatus_F/1
  BCM_RearWiperStatus_S/1 -> BCM_RearWiperStatuscv/1
  BCM_RearWiperStatus_L/1 -> BCM_RearWiperStatus_S/1
  BCM_RearWiperStatus_Convert/1 -> BCM_RearWiperStatus_L/1
  BCM_RearWiperStatus_Sub/1(Out1) -> BCM_RearWiperStatus_Convert/1
  BCM_RearWiperStatus_sat/1 -> BCM_RearWiperStatus_Out/1
  BCM_RearWiperStatus_Ad/1 -> BCM_RearWiperStatus_sat/1
  BCM_RearWiperStatus_O/1 -> BCM_RearWiperStatus_Ad/2
  BCM_RearWiperStatus_F/1 -> BCM_RearWiperStatus_Ad/1
  BCM_PowerStatusFeedbackcv/1 -> BCM_PowerStatusFeedback_F/1
  BCM_PowerStatusFeedback_S/1 -> BCM_PowerStatusFeedbackcv/1
  BCM_PowerStatusFeedback_L/1 -> BCM_PowerStatusFeedback_S/1
  BCM_PowerStatusFeedback_Convert/1 -> BCM_PowerStatusFeedback_L/1
  BCM_PowerStatusFeedback_Sub/1(Out1) -> BCM_PowerStatusFeedback_Convert/1
  BCM_PowerStatusFeedback_sat/1 -> BCM_PowerStatusFeedback_Out/1
  BCM_PowerStatusFeedback_Ad/1 -> BCM_PowerStatusFeedback_sat/1
  BCM_PowerStatusFeedback_O/1 -> BCM_PowerStatusFeedback_Ad/2
  BCM_PowerStatusFeedback_F/1 -> BCM_PowerStatusFeedback_Ad/1
  BCM_DriverDoorLockStatuscv/1 -> BCM_DriverDoorLockStatus_F/1
  BCM_DriverDoorLockStatus_S/1 -> BCM_DriverDoorLockStatuscv/1
  BCM_DriverDoorLockStatus_L/1 -> BCM_DriverDoorLockStatus_S/1
  BCM_DriverDoorLockStatus_Convert/1 -> BCM_DriverDoorLockStatus_L/1
  BCM_DriverDoorLockStatus_Sub/1(Out1) -> BCM_DriverDoorLockStatus_Convert/1
  Demux/6 -> BCM_PowerStatusFeedback_Sub/1(In1), BCM_DriverDoorLockStatus_Sub/1(In1), BCM_RearWiperStatus_Sub/1(In1), BCM_FrontWiperStatus_Sub/1(In1)
  BCM_DriverDoorLockStatus_sat/1 -> BCM_DriverDoorLockStatus_Out/1
  BCM_DriverDoorLockStatus_Ad/1 -> BCM_DriverDoorLockStatus_sat/1
  BCM_DriverDoorLockStatus_O/1 -> BCM_DriverDoorLockStatus_Ad/2
  BCM_DriverDoorLockStatus_F/1 -> BCM_DriverDoorLockStatus_Ad/1
  BCM_emergencylightstatuscv/1 -> BCM_emergencylightstatus_F/1
  BCM_emergencylightstatus_S/1 -> BCM_emergencylightstatuscv/1
  BCM_emergencylightstatus_L/1 -> BCM_emergencylightstatus_S/1
  BCM_emergencylightstatus_Convert/1 -> BCM_emergencylightstatus_L/1
  BCM_emergencylightstatus_Sub/1(Out1) -> BCM_emergencylightstatus_Convert/1
  BCM_emergencylightstatus_sat/1 -> BCM_emergencylightstatus_Out/1
  BCM_emergencylightstatus_Ad/1 -> BCM_emergencylightstatus_sat/1
  BCM_emergencylightstatus_O/1 -> BCM_emergencylightstatus_Ad/2
  BCM_emergencylightstatus_F/1 -> BCM_emergencylightstatus_Ad/1
  BCM_PassengerDoorLockStatuscv/1 -> BCM_PassengerDoorLockStatus_F/1
  BCM_PassengerDoorLockStatus_S/1 -> BCM_PassengerDoorLockStatuscv/1
  BCM_PassengerDoorLockStatus_L/1 -> BCM_PassengerDoorLockStatus_S/1
  BCM_PassengerDoorLockStatus_Convert/1 -> BCM_PassengerDoorLockStatus_L/1
  BCM_PassengerDoorLockStatus_Sub/1(Out1) -> BCM_PassengerDoorLockStatus_Convert/1
  Demux/5 -> BCM_PassengerDoorLockStatus_Sub/1(In1), BCM_emergencylightstatus_Sub/1(In1)
  BCM_PassengerDoorLockStatus_sat/1 -> BCM_PassengerDoorLockStatus_Out/1
  BCM_PassengerDoorLockStatus_Ad/1 -> BCM_PassengerDoorLockStatus_sat/1
  BCM_PassengerDoorLockStatus_O/1 -> BCM_PassengerDoorLockStatus_Ad/2
  BCM_PassengerDoorLockStatus_F/1 -> BCM_PassengerDoorLockStatus_Ad/1
  BCM_DriverDoorStatuscv/1 -> BCM_DriverDoorStatus_F/1
  BCM_DriverDoorStatus_S/1 -> BCM_DriverDoorStatuscv/1
  BCM_DriverDoorStatus_L/1 -> BCM_DriverDoorStatus_S/1
  BCM_DriverDoorStatus_Convert/1 -> BCM_DriverDoorStatus_L/1
  BCM_DriverDoorStatus_Sub/1(Out1) -> BCM_DriverDoorStatus_Convert/1
  BCM_DriverDoorStatus_sat/1 -> BCM_DriverDoorStatus_Out/1
  BCM_DriverDoorStatus_Ad/1 -> BCM_DriverDoorStatus_sat/1
  BCM_DriverDoorStatus_O/1 -> BCM_DriverDoorStatus_Ad/2
  BCM_DriverDoorStatus_F/1 -> BCM_DriverDoorStatus_Ad/1
  BCM_PassengerDoorStatuscv/1 -> BCM_PassengerDoorStatus_F/1
  BCM_PassengerDoorStatus_S/1 -> BCM_PassengerDoorStatuscv/1
  BCM_PassengerDoorStatus_L/1 -> BCM_PassengerDoorStatus_S/1
  BCM_PassengerDoorStatus_Convert/1 -> BCM_PassengerDoorStatus_L/1
  BCM_PassengerDoorStatus_Sub/1(Out1) -> BCM_PassengerDoorStatus_Convert/1
  BCM_PassengerDoorStatus_sat/1 -> BCM_PassengerDoorStatus_Out/1
  BCM_PassengerDoorStatus_Ad/1 -> BCM_PassengerDoorStatus_sat/1
  BCM_PassengerDoorStatus_O/1 -> BCM_PassengerDoorStatus_Ad/2
  BCM_PassengerDoorStatus_F/1 -> BCM_PassengerDoorStatus_Ad/1
  BCM_LeftRearDoorStatuscv/1 -> BCM_LeftRearDoorStatus_F/1
  BCM_LeftRearDoorStatus_S/1 -> BCM_LeftRearDoorStatuscv/1
  BCM_LeftRearDoorStatus_L/1 -> BCM_LeftRearDoorStatus_S/1
  BCM_LeftRearDoorStatus_Convert/1 -> BCM_LeftRearDoorStatus_L/1
  BCM_LeftRearDoorStatus_Sub/1(Out1) -> BCM_LeftRearDoorStatus_Convert/1
  BCM_LeftRearDoorStatus_sat/1 -> BCM_LeftRearDoorStatus_Out/1
  BCM_LeftRearDoorStatus_Ad/1 -> BCM_LeftRearDoorStatus_sat/1
  BCM_LeftRearDoorStatus_O/1 -> BCM_LeftRearDoorStatus_Ad/2
  BCM_LeftRearDoorStatus_F/1 -> BCM_LeftRearDoorStatus_Ad/1
  BCM_RightRearDoorStatuscv/1 -> BCM_RightRearDoorStatus_F/1
  BCM_RightRearDoorStatus_S/1 -> BCM_RightRearDoorStatuscv/1
  BCM_RightRearDoorStatus_L/1 -> BCM_RightRearDoorStatus_S/1
  BCM_RightRearDoorStatus_Convert/1 -> BCM_RightRearDoorStatus_L/1
  BCM_RightRearDoorStatus_Sub/1(Out1) -> BCM_RightRearDoorStatus_Convert/1
  BCM_RightRearDoorStatus_sat/1 -> BCM_RightRearDoorStatus_Out/1
  BCM_RightRearDoorStatus_Ad/1 -> BCM_RightRearDoorStatus_sat/1
  BCM_RightRearDoorStatus_O/1 -> BCM_RightRearDoorStatus_Ad/2
  BCM_RightRearDoorStatus_F/1 -> BCM_RightRearDoorStatus_Ad/1
  BCM_TrunkDoorStatuscv/1 -> BCM_TrunkDoorStatus_F/1
  BCM_TrunkDoorStatus_S/1 -> BCM_TrunkDoorStatuscv/1
  BCM_TrunkDoorStatus_L/1 -> BCM_TrunkDoorStatus_S/1
  BCM_TrunkDoorStatus_Convert/1 -> BCM_TrunkDoorStatus_L/1
  BCM_TrunkDoorStatus_Sub/1(Out1) -> BCM_TrunkDoorStatus_Convert/1
  BCM_TrunkDoorStatus_sat/1 -> BCM_TrunkDoorStatus_Out/1
  BCM_TrunkDoorStatus_Ad/1 -> BCM_TrunkDoorStatus_sat/1
  BCM_TrunkDoorStatus_O/1 -> BCM_TrunkDoorStatus_Ad/2
  BCM_TrunkDoorStatus_F/1 -> BCM_TrunkDoorStatus_Ad/1
  BCM_HoodStatuscv/1 -> BCM_HoodStatus_F/1
  BCM_HoodStatus_S/1 -> BCM_HoodStatuscv/1
  BCM_HoodStatus_L/1 -> BCM_HoodStatus_S/1
  BCM_HoodStatus_Convert/1 -> BCM_HoodStatus_L/1
  BCM_HoodStatus_Sub/1(Out1) -> BCM_HoodStatus_Convert/1
  Demux/3 -> BCM_DriverDoorStatus_Sub/1(In1), BCM_HoodStatus_Sub/1(In1), BCM_PassengerDoorStatus_Sub/1(In1), BCM_RightRearDoorStatus_Sub/1(In1), BCM_TrunkDoorStatus_Sub/1(In1), BCM_LeftRearDoorStatus_Sub/1(In1)
  BCM_HoodStatus_sat/1 -> BCM_HoodStatus_Out/1
  BCM_HoodStatus_Ad/1 -> BCM_HoodStatus_sat/1
  BCM_HoodStatus_O/1 -> BCM_HoodStatus_Ad/2
  BCM_HoodStatus_F/1 -> BCM_HoodStatus_Ad/1
  BCM_TurnIndicatorLeftcv/1 -> BCM_TurnIndicatorLeft_F/1
  BCM_TurnIndicatorLeft_S/1 -> BCM_TurnIndicatorLeftcv/1
  BCM_TurnIndicatorLeft_L/1 -> BCM_TurnIndicatorLeft_S/1
  BCM_TurnIndicatorLeft_Convert/1 -> BCM_TurnIndicatorLeft_L/1
  BCM_TurnIndicatorLeft_Sub/1(Out1) -> BCM_TurnIndicatorLeft_Convert/1
  BCM_TurnIndicatorLeft_sat/1 -> BCM_TurnIndicatorLeft_Out/1
  BCM_TurnIndicatorLeft_Ad/1 -> BCM_TurnIndicatorLeft_sat/1
  BCM_TurnIndicatorLeft_O/1 -> BCM_TurnIndicatorLeft_Ad/2
  BCM_TurnIndicatorLeft_F/1 -> BCM_TurnIndicatorLeft_Ad/1
  BCM_TurnIndicatorRightcv/1 -> BCM_TurnIndicatorRight_F/1
  BCM_TurnIndicatorRight_S/1 -> BCM_TurnIndicatorRightcv/1
  BCM_TurnIndicatorRight_L/1 -> BCM_TurnIndicatorRight_S/1
  BCM_TurnIndicatorRight_Convert/1 -> BCM_TurnIndicatorRight_L/1
  BCM_TurnIndicatorRight_Sub/1(Out1) -> BCM_TurnIndicatorRight_Convert/1
  BCM_TurnIndicatorRight_sat/1 -> BCM_TurnIndicatorRight_Out/1
  BCM_TurnIndicatorRight_Ad/1 -> BCM_TurnIndicatorRight_sat/1
  BCM_TurnIndicatorRight_O/1 -> BCM_TurnIndicatorRight_Ad/2
  BCM_TurnIndicatorRight_F/1 -> BCM_TurnIndicatorRight_Ad/1
  BCM_FrontWashStatuscv/1 -> BCM_FrontWashStatus_F/1
  BCM_FrontWashStatus_S/1 -> BCM_FrontWashStatuscv/1
  BCM_FrontWashStatus_L/1 -> BCM_FrontWashStatus_S/1
  BCM_FrontWashStatus_Convert/1 -> BCM_FrontWashStatus_L/1
  BCM_FrontWashStatus_Sub/1(Out1) -> BCM_FrontWashStatus_Convert/1
  Demux/2 -> BCM_FrontWashStatus_Sub/1(In1), BCM_TurnIndicatorLeft_Sub/1(In1), BCM_TurnIndicatorRight_Sub/1(In1)
  BCM_FrontWashStatus_sat/1 -> BCM_FrontWashStatus_Out/1
  BCM_FrontWashStatus_Ad/1 -> BCM_FrontWashStatus_sat/1
  BCM_FrontWashStatus_O/1 -> BCM_FrontWashStatus_Ad/2
  BCM_FrontWashStatus_F/1 -> BCM_FrontWashStatus_Ad/1
  Demux/1 -> ?
